simulink subsystem "cvrs_contractility_control"  (R2020b)
settings: Solver=VariableStepAuto  StartTime=0.0  StopTime=10.0  RelTol=1e-3
settings Model: Creator=RH  LastModifiedBy=Marco

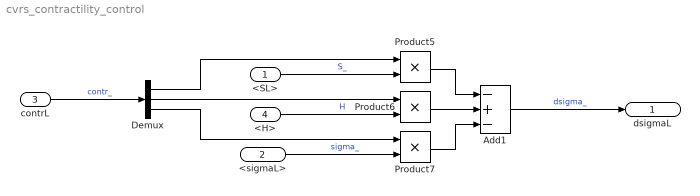
== system cvrs_contractility_control ==
  <SL> : Inport
  <sigmaL> : Inport  Port=2
  contrL : Inport  Port=3  OutDataTypeStr=double  PortDimensions=3
  <H> : Inport  Port=4
  Add1 : Sum  Inputs=-+-
  Demux : Demux  Outputs=3
  Product5 : Product
  Product6 : Product
  Product7 : Product
  dsigmaL : Outport
  wires:
  <SL>/1 -> Product5/2  "S_"
  Add1/1 -> dsigmaL/1  "dsigma_"
  Demux/3 -> Product7/1
  Product7/1 -> Add1/3
  Demux/2 -> Product6/1
  contrL/1 -> Demux/1  "contr_"
  Product5/1 -> Add1/1
  Demux/1 -> Product5/1
  <sigmaL>/1 -> Product7/2  "sigma_"
  Product6/1 -> Add1/2
  <H>/1 -> Product6/2  "H"
